simulink model "TrqBasedOnEfficient"  (R2022b)
settings: Solver=VariableStepAuto  StartTime=0.0  StopTime=120  RelTol=1e-3
libraries: Solver_SF x1, simulink x1
settings Model: Creator=12045  LastModifiedBy=12045
settings DebuggingCC: ParameterPrecisionLossMsg=none

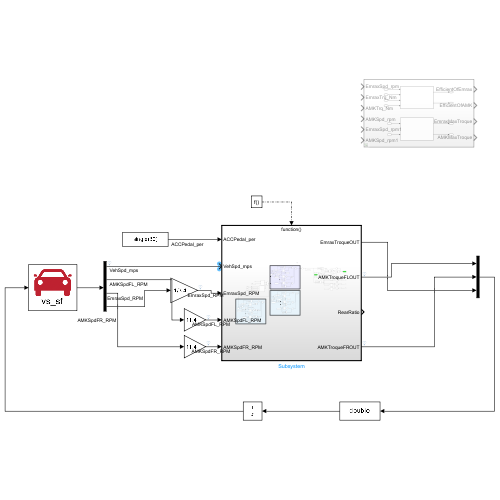
[thumbnail: Simulink's stored preview of the top-level diagram]
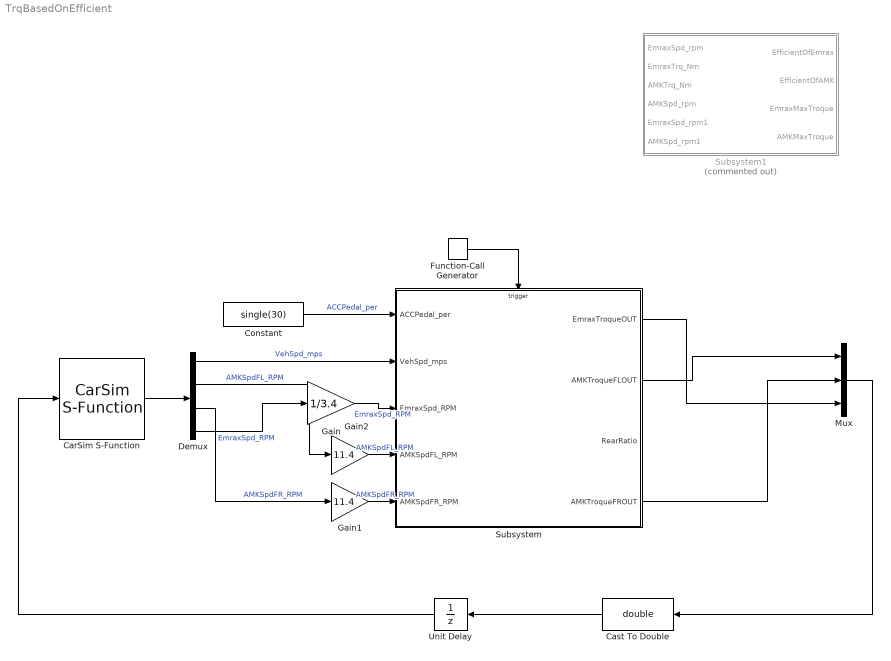
== system TrqBasedOnEfficient ==
  CarSim S-Function : Solver_SF/CarSim S-Function  Priority=1  SIMFILE=simfile.sim  Run_RTs=off  vs_state_ind=Run  StopMode_ind=Vehicle Model
  Cast To Double : DataTypeConversion  OutDataTypeStr=double  SaturateOnIntegerOverflow=off  RndMeth=Floor
  Constant : Constant  Value=single(30)
  Demux : Demux
  Function-Call Generator : simulink/Ports & Subsystems/Function-Call Generator  sample_time=0.01  numberOfIterations=1  DisallowWideOutput=off
  Gain : Gain  Gain=1/3.4
  Gain1 : Gain  Gain=11.4
  Gain2 : Gain  Gain=11.4
  Mux : Mux  Inputs=3
  Subsystem : Subsystem
  Subsystem1 : Subsystem  Commented=on
  Unit Delay : UnitDelay  SampleTime=-1  HasFrameUpgradeWarning=on
  wires:
  Function-Call Generator/1 -> Subsystem/Trigger
  CarSim S-Function/1 -> Demux/1
  Demux/1 -> Subsystem/2(VehSpd_mps)  "VehSpd_mps"
  Demux/2 -> Gain2/1  "AMKSpdFL_RPM"
  Demux/3 -> Gain1/1  "AMKSpdFR_RPM"
  Demux/4 -> Gain/1  "EmraxSpd_RPM"
  Constant/1 -> Subsystem/1(ACCPedal_per)  "ACCPedal_per"
  Subsystem/2(AMKTroqueFLOUT) -> Mux/1
  Subsystem/1(EmraxTroqueOUT) -> Mux/3
  Subsystem/4(AMKTroqueFROUT) -> Mux/2
  Mux/1 -> Cast To Double/1
  Unit Delay/1 -> CarSim S-Function/1
  Cast To Double/1 -> Unit Delay/1
  Gain/1 -> Subsystem/3(EmraxSpd_RPM)  "EmraxSpd_RPM"
  Gain1/1 -> Subsystem/5(AMKSpdFR_RPM)  "AMKSpdFR_RPM"
  Gain2/1 -> Subsystem/4(AMKSpdFL_RPM)  "AMKSpdFL_RPM"

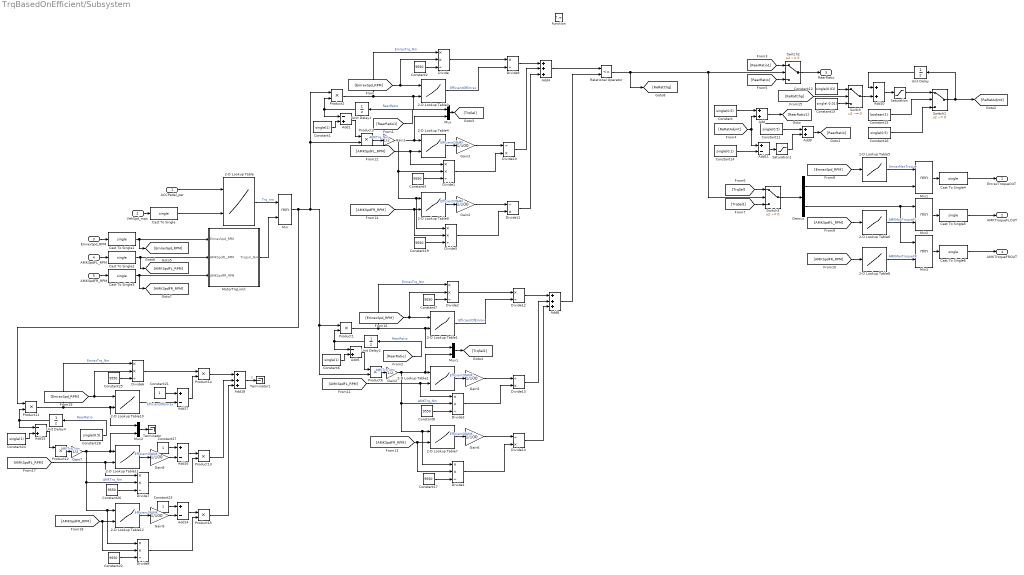
== system TrqBasedOnEfficient/Subsystem ==
  ACCPedal_per : Inport
  VehSpd_mps : Inport  Port=2
  EmraxSpd_RPM : Inport  Port=3
  AMKSpdFL_RPM : Inport  Port=4
  AMKSpdFR_RPM : Inport  Port=5
  function : TriggerPort  TriggerType=function-call  VariantControl=(inherit)
  2-D Lookup Table : Lookup_n-D  BreakpointsForDimension1=single([0 10 20 30 40 50 60 70 80 90 100])  BreakpointsForDimension2=single([5.40000009536743 10.8000001907349 16.2000007629395 21.6000003814697 27 32.4000015258789 37.7999992370605 43.2000007629395 48.5999984741211 54 59.4000015258789 64.8000030517578 70.1999969482422 75.5999984741211 81 86.4000015258789 91.8000030517578 97.1999969482422 102.599998474121 108])  BreakpointsForDimension1DataTypeStr=single  BreakpointsForDimension2DataTypeStr=single  Table=single([0 0 0 0 0 0 0 0 0 0 0 0 0 0 0 0 0 0 0 0;20 20 20 20 20 20 20 18 18 18 17 17 16 16 15 15 15 14 14 14;35 35 35 35 35 35 30 30 25 25 25 25 20 20 20 20 20 20 20 18;50 50 50 50 50 50 50 50 50 40 40 40 40 40 40 40 40 40 38 35;79 79 79 79 85 85 85 90 95 100 110 110 110 100 90 90 80 72 70 65;100 100 100 105 105 105 110 110 110 110 115 115 125 125 120 110 90 80 76 70;120 120 120 120 125 125 125 135 135 135 135 135 135 130 130 120 100 90 82 74;125 125 125 130 135 140 145 155 155 155 155 155 155 155 155 135 110 100 88 82;130 160 160 160 160 170 160 160 160 160 160 160 160 160 160 142 120 105 94 88;130 160 160 160 160 170 160 160 160 160 160 160 160 160 160 142 120 105 95 91;170 170 180 180 180 210 200 200 200 200 200 200 190 180 180 152 133 118 106 100])  InternalRulePriority=Speed  RndMeth=Simplest
      settings: InputPortMap=u0,u1
  2-D Lookup Table1 : Lookup_n-D  BreakpointsForDimension1=[0;200;400;600;800;1000;1200;1400;1600;1800;2000;2200;2400;2600;2800;3000;3200;3400;3600;3800;4000;4200;4400;4600;4800;5000;5200;5400]  BreakpointsForDimension2=[0;25;50;75;100;125;150;175;200;225;250]  Table=[0.7 0.7 0.7 0.7 0.7 0.7 0.7 0.7 0.7 0.7 0.7;0.7 0.7 0.7 0.7 0.7 0.7 0.7 0.7 0.7 0.7 0.7;0.7 0.7 0.86 0.86 0.86 0.86 0.86 0.7 0.7 0.7 0.7;0.7 0.7 0.86 0.86 0.86 0.86 0.86 0.86 0.7 0.7 0.7;0.7 0.82 0.86 0.9 0.9 0.9 0.86 0.86 0.86 0.7 0.7;0.7 0.82 0.86 0.9 0.9 0.9 0.9 0.9 0.86 0.86 0.7;0.7 0.7 0.9 0.94 0.94 0.94 0.94 0.9 0.9 0.86 0.7;0.7 0.82 0.9 0.94 0.94 0.95 0.95 0.94 0.9 0.9 0.7;0.7 0.86 0.9 0.94 0.95 0.95 0.95 0.94 0.9 0.9 0.7;0.7 0.86 0.9 0.94 0.96 0.98 0.95 0.94 0.9 0.9 0.7;0.7 0.86 0.9 0.95 0.96 0.96 0.95 0.94 0.9 0.9 0.7;0.7 0.86 0.9 0.95 0.96 0.96 0.95 0.94 0.94 0.9 0.7;0.7 0.86 0.9 0.95 0.96 0.96 0.95 0.94 0.94 0.9 0.7;0.7 0.86 0.9 0.95 0.96 0.96 0.95 0.94 0.94 0.9 0.7;0.7 0.86 0.9 0.95 0.96 0.96 0.95 0.94 0.94 0.9 0.7;0.7 0.86 0.9 0.95 0.96 0.96 0.95 0.94 0.94 0.9 0.7;0.7 0.86 0.9 0.95 0.96 0.96 0.95 0.94 0.94 0.9 0.7;0.7 0.86 0.9 0.94 0.96 0.96 0.95 0.94 0.94 0.9 0.7;0.7 0.86 0.9 0.94 0.96 0.95 0.95 0.94 0.94 0.9 0.7;0.7 0.86 0.9 0.94 0.96 0.95 0.95 0.94 0.94 0.9 0.7;0.7 0.86 0.9 0.94 0.95 0.95 0.95 0.94 0.94 0.9 0.7;0.7 0.7 0.9 0.94 0.95 0.95 0.95 0.94 0.94 0.9 0.7;0.7 0.7 0.86 0.94 0.94 0.95 0.95 0.94 0.94 0.9 0.7;0.7 0.7 0.86 0.9 0.94 0.95 0.95 0.94 0.94 0.9 0.7;0.7 0.7 0.7 0.9 0.94 0.94 0.94 0.94 0.94 0.9 0.7;0.7 0.7 0.7 0.86 0.9 0.94 0.94 0.94 0.94 0.9 0.7;0.7 0.7 0.7 0.86 0.9 0.9 0.94 0.94 0.94 0.9 0.7;0.7 0.7 0.7 0.86 0.9 0.9 0.94 0.94 0.94 0.9 0.7]  InternalRulePriority=Speed  RndMeth=Simplest
      settings: InputPortMap=u0,u1
  2-D Lookup Table10 : Lookup_n-D  BreakpointsForDimension1=[0;200;400;600;800;1000;1200;1400;1600;1800;2000;2200;2400;2600;2800;3000;3200;3400;3600;3800;4000;4200;4400;4600;4800;5000;5200;5400]  BreakpointsForDimension2=[0;25;50;75;100;125;150;175;200;225;250]  Table=[0.7 0.7 0.7 0.7 0.7 0.7 0.7 0.7 0.7 0.7 0.7;0.7 0.7 0.7 0.7 0.7 0.7 0.7 0.7 0.7 0.7 0.7;0.7 0.7 0.86 0.86 0.86 0.86 0.86 0.7 0.7 0.7 0.7;0.7 0.7 0.86 0.86 0.86 0.86 0.86 0.86 0.7 0.7 0.7;0.7 0.82 0.86 0.9 0.9 0.9 0.86 0.86 0.86 0.7 0.7;0.7 0.82 0.86 0.9 0.9 0.9 0.9 0.9 0.86 0.86 0.7;0.7 0.7 0.9 0.94 0.94 0.94 0.94 0.9 0.9 0.86 0.7;0.7 0.82 0.9 0.94 0.94 0.95 0.95 0.94 0.9 0.9 0.7;0.7 0.86 0.9 0.94 0.95 0.95 0.95 0.94 0.9 0.9 0.7;0.7 0.86 0.9 0.94 0.96 0.98 0.95 0.94 0.9 0.9 0.7;0.7 0.86 0.9 0.95 0.96 0.96 0.95 0.94 0.9 0.9 0.7;0.7 0.86 0.9 0.95 0.96 0.96 0.95 0.94 0.94 0.9 0.7;0.7 0.86 0.9 0.95 0.96 0.96 0.95 0.94 0.94 0.9 0.7;0.7 0.86 0.9 0.95 0.96 0.96 0.95 0.94 0.94 0.9 0.7;0.7 0.86 0.9 0.95 0.96 0.96 0.95 0.94 0.94 0.9 0.7;0.7 0.86 0.9 0.95 0.96 0.96 0.95 0.94 0.94 0.9 0.7;0.7 0.86 0.9 0.95 0.96 0.96 0.95 0.94 0.94 0.9 0.7;0.7 0.86 0.9 0.94 0.96 0.96 0.95 0.94 0.94 0.9 0.7;0.7 0.86 0.9 0.94 0.96 0.95 0.95 0.94 0.94 0.9 0.7;0.7 0.86 0.9 0.94 0.96 0.95 0.95 0.94 0.94 0.9 0.7;0.7 0.86 0.9 0.94 0.95 0.95 0.95 0.94 0.94 0.9 0.7;0.7 0.7 0.9 0.94 0.95 0.95 0.95 0.94 0.94 0.9 0.7;0.7 0.7 0.86 0.94 0.94 0.95 0.95 0.94 0.94 0.9 0.7;0.7 0.7 0.86 0.9 0.94 0.95 0.95 0.94 0.94 0.9 0.7;0.7 0.7 0.7 0.9 0.94 0.94 0.94 0.94 0.94 0.9 0.7;0.7 0.7 0.7 0.86 0.9 0.94 0.94 0.94 0.94 0.9 0.7;0.7 0.7 0.7 0.86 0.9 0.9 0.94 0.94 0.94 0.9 0.7;0.7 0.7 0.7 0.86 0.9 0.9 0.94 0.94 0.94 0.9 0.7]  InternalRulePriority=Speed  RndMeth=Simplest
      settings: InputPortMap=u0,u1
  2-D Lookup Table{2,4,7,9,11..12} (6 alike) : Lookup_n-D  BreakpointsForDimension1=[1.3;2.7;5.4;7.9;10.4;12.5;14.4;16;17.4;18.5;19.6]  BreakpointsForDimension2=[500;1000;2000;3000;4000;6000;10000;12000;15000;19000]  Table=[64.37 71.33 73.64 74.7 75.43 76.57 77 77.08 77.56 78.14;58.42 70.48 77.57 80.4 82.01 83.92 85.16 85.44 85.97 86.5;44.94 60.81 73.35 78.82 81.94 85.43 88.2 88.88 89.71 90.44;35.59 51.9 67.02 74.26 78.54 83.42 87.58 88.65 89.84 90.86;29.14 44.78 61.01 69.41 74.57 80.62 85.93 87.34 88.86 90.16;24.17 38.71 55.22 64.39 70.24 77.3 83.73 85.48 87.37 88.98;20.41 33.76 50.04 59.65 65.99 73.88 81.33 83.42 85.66 87.59;17.31 29.4 45.1 54.87 61.55 70.1 78.56 80.97 83.56 85.81;14.82 25.75 40.67 50.41 57.28 66.34 75.7 78.4 81.34 83.91;12.81 22.67 36.72 46.3 53.25 62.67 72.77 75.75 79.02 81.91;11.17 20.05 33.21 42.51 49.44 59.09 69.82 73.06 76.63 79.83]  InternalRulePriority=Speed  RndMeth=Simplest
      settings: InputPortMap=u0,u1
  2-D Lookup Table3 : Lookup_n-D  BreakpointsForDimension1=[0;200;400;600;800;1000;1200;1400;1600;1800;2000;2200;2400;2600;2800;3000;3200;3400;3600;3800;4000;4200;4400;4600;4800;5000;5200;5400]  BreakpointsForDimension2=[0;25;50;75;100;125;150;175;200;225;250]  Table=[0.7 0.7 0.7 0.7 0.7 0.7 0.7 0.7 0.7 0.7 0.7;0.7 0.7 0.7 0.7 0.7 0.7 0.7 0.7 0.7 0.7 0.7;0.7 0.7 0.86 0.86 0.86 0.86 0.86 0.7 0.7 0.7 0.7;0.7 0.7 0.86 0.86 0.86 0.86 0.86 0.86 0.7 0.7 0.7;0.7 0.82 0.86 0.9 0.9 0.9 0.86 0.86 0.86 0.7 0.7;0.7 0.82 0.86 0.9 0.9 0.9 0.9 0.9 0.86 0.86 0.7;0.7 0.7 0.9 0.94 0.94 0.94 0.94 0.9 0.9 0.86 0.7;0.7 0.82 0.9 0.94 0.94 0.95 0.95 0.94 0.9 0.9 0.7;0.7 0.86 0.9 0.94 0.95 0.95 0.95 0.94 0.9 0.9 0.7;0.7 0.86 0.9 0.94 0.96 0.98 0.95 0.94 0.9 0.9 0.7;0.7 0.86 0.9 0.95 0.96 0.96 0.95 0.94 0.9 0.9 0.7;0.7 0.86 0.9 0.95 0.96 0.96 0.95 0.94 0.94 0.9 0.7;0.7 0.86 0.9 0.95 0.96 0.96 0.95 0.94 0.94 0.9 0.7;0.7 0.86 0.9 0.95 0.96 0.96 0.95 0.94 0.94 0.9 0.7;0.7 0.86 0.9 0.95 0.96 0.96 0.95 0.94 0.94 0.9 0.7;0.7 0.86 0.9 0.95 0.96 0.96 0.95 0.94 0.94 0.9 0.7;0.7 0.86 0.9 0.95 0.96 0.96 0.95 0.94 0.94 0.9 0.7;0.7 0.86 0.9 0.94 0.96 0.96 0.95 0.94 0.94 0.9 0.7;0.7 0.86 0.9 0.94 0.96 0.95 0.95 0.94 0.94 0.9 0.7;0.7 0.86 0.9 0.94 0.96 0.95 0.95 0.94 0.94 0.9 0.7;0.7 0.86 0.9 0.94 0.95 0.95 0.95 0.94 0.94 0.9 0.7;0.7 0.7 0.9 0.94 0.95 0.95 0.95 0.94 0.94 0.9 0.7;0.7 0.7 0.86 0.94 0.94 0.95 0.95 0.94 0.94 0.9 0.7;0.7 0.7 0.86 0.9 0.94 0.95 0.95 0.94 0.94 0.9 0.7;0.7 0.7 0.7 0.9 0.94 0.94 0.94 0.94 0.94 0.9 0.7;0.7 0.7 0.7 0.86 0.9 0.94 0.94 0.94 0.94 0.9 0.7;0.7 0.7 0.7 0.86 0.9 0.9 0.94 0.94 0.94 0.9 0.7;0.7 0.7 0.7 0.86 0.9 0.9 0.94 0.94 0.94 0.9 0.7]  InternalRulePriority=Speed  RndMeth=Simplest
      settings: InputPortMap=u0,u1
  2-D Lookup Table5 : Lookup_n-D  NumberOfTableDimensions=1  BreakpointsForDimension1=[200;400;600;800;1000;1200;1400;1600;1800;2000;2200;2400;2600;2800;3000;3200;3400;3600;3800;4000;4200;4400;4600;4800;5000;5200;5400]  BreakpointsForDimension2=[1:3]  Table=[229.85;229.85;229.85;229.85;229.85;229.85;229.85;229.85;229.85;229.85;229.85;229.85;229.46;229.16;228.86;228.86;228.86;228.86;228.86;227.86;227.86;226.87;225.86;224.86;220.86;218.87;215.87]  InternalRulePriority=Speed  RndMeth=Simplest
  2-D Lookup Table6 : Lookup_n-D  NumberOfTableDimensions=1  BreakpointsForDimension1=[0;1000;2000;3000;4000;5000;6000;7000;8000;9000;10000;11000;12000;13000;14000;15000;16000;17000;18000;19000]  BreakpointsForDimension2=[1:3]  Table=[21;21;21;21;21;21;21;21;21;21;21;21;21;21;20;17.5;15;12.5;8;0]  InternalRulePriority=Speed  RndMeth=Simplest
  2-D Lookup Table8 : Lookup_n-D  NumberOfTableDimensions=1  BreakpointsForDimension1=[0;1000;2000;3000;4000;5000;6000;7000;8000;9000;10000;11000;12000;13000;14000;15000;16000;17000;18000;19000]  BreakpointsForDimension2=[1:3]  Table=[21;21;21;21;21;21;21;21;21;21;21;21;21;21;20;17.5;15;12.5;8;0]  InternalRulePriority=Speed  RndMeth=Simplest
  Add : Sum
  Add1 : Sum  Inputs=-+
  Add10 : Sum
  Add{11,14,16..17} (4 alike) : Sum  Inputs=+-
  Add15 : Sum  Inputs=-+
  Add18 : Sum  Inputs=+++
  Add4 : Sum  Inputs=+++
  Add5 : Sum  Inputs=-+
  Add8 : Sum  Inputs=+++
  Add9 : Sum
  Cast To Single{,1..6} (7 alike) : DataTypeConversion  OutDataTypeStr=single  SaturateOnIntegerOverflow=off  RndMeth=Floor
  Constant{,11,16,28} (4 alike) : Constant  Value=single(0.5)
  Constant1 : Constant  Value=single(1)
  Constant12 : Constant  Value=single(0.01)
  Constant13 : Constant  Value=single(-0.01)
  Constant14 : Constant  Value=single(0.1)
  Constant15 : Constant  Value=boolean(1)
  Constant{2..3,7..8,17,19,22,25..26} (9 alike) : Constant  Value=9550
  Constant21 : Constant
  Constant23 : Constant
  Constant24 : Constant  Value=single(1)
  Constant27 : Constant
  Constant6 : Constant  Value=single(1)
  Demux : Demux  Outputs=2
  Divide{,1..8} (9 alike) : Product  Inputs=**/
  Divide{10..11,13..14} (4 alike) : Product  Inputs=/*
  Divide12 : Product  Inputs=*/
  Divide9 : Product  Inputs=*/
  Gain1 : Gain  Gain=1/2
  Gain2 : Gain  Gain=1/2
  Gain{3..6,8..9} (6 alike) : Gain  Gain=1/100
  Gain7 : Gain  Gain=1/2
  Min{,1..3} (4 alike) : MinMax  Inputs=2
  MotorTrqLimit : Subsystem
  Mux : Mux  Inputs=2
  Mux1 : Mux  Inputs=2
  Mux2 : Mux  Inputs=2
  Product{1..3,6,11..15} (9 alike) : Product
  Relational Operator : RelationalOperator  Operator=<=  OutDataTypeStr=boolean  RndMeth=Simplest  InputSameDT=off
  Saturation : Saturate  LowerLimit=0
  Saturation1 : Saturate  UpperLimit=1  LowerLimit=0.5
  Switch{,1..3} (4 alike) : Switch  Criteria=u2 ~= 0  SaturateOnIntegerOverflow=off  InputSameDT=off
  Terminator : Terminator
  Terminator1 : Terminator
  Unit Delay : UnitDelay  SampleTime=-1  HasFrameUpgradeWarning=on
  Unit Delay1 : UnitDelay  InitialCondition=0.5  SampleTime=-1  HasFrameUpgradeWarning=on
  Unit Delay2 : UnitDelay  InitialCondition=0.5  SampleTime=-1  HasFrameUpgradeWarning=on
  Unit Delay4 : UnitDelay  InitialCondition=0.5  SampleTime=-1  HasFrameUpgradeWarning=on
  EmraxTroqueOUT : Outport
  AMKTroqueFLOUT : Outport  Port=2
  RearRatio : Outport  Port=3
  AMKTroqueFROUT : Outport  Port=4
  wires:
  2-D Lookup Table/1 -> Min/1  "Trq_nm"
  MotorTrqLimit/1(TrqLim_Nm) -> Min/2
  2-D Lookup Table6/1 -> Min2/2  "AMKMaxTroqueFL"
  [EmraxSpd_RPM] -> 2-D Lookup Table5/1
  [AMKSpdFL_RPM] -> 2-D Lookup Table6/1
  2-D Lookup Table5/1 -> Min1/1  "EmraxMaxTroque"
  ACCPedal_per/1 -> 2-D Lookup Table/1
  EmraxSpd_RPM/1 -> Cast To Single1/1
  VehSpd_mps/1 -> Cast To Single/1
  Unit Delay1/1 -> Add1/1, Product2/2
  [AMKSpdFL_RPM] -> Divide1/1, 2-D Lookup Table4/2
  [EmraxSpd_RPM] -> Divide/2, 2-D Lookup Table3/1
  2-D Lookup Table4/1 -> Gain3/1  "EfficientOfAMK"
  2-D Lookup Table3/1 -> Divide9/2  "EfficientOfEmrax"
  Constant1/1 -> Add1/2
  Product3/1 -> Gain1/1  "AMKTrq_Nm"
  [RearRatio1] -> Unit Delay1/1  "RearRatio"
  Add1/1 -> Product3/1
  Min/1 -> Product11/1, Product6/2, Product1/1, Product2/1, Product3/2
  Product2/1 -> Divide/1, Mux/1, 2-D Lookup Table3/2  "EmraxTrq_Nm"
  Constant2/1 -> Divide/3
  Constant3/1 -> Divide1/3
  Divide1/1 -> Divide10/2
  Divide/1 -> Divide9/1
  Divide9/1 -> Add4/1
  Divide10/1 -> Add4/2
  Divide13/1 -> Add8/2
  Divide12/1 -> Add8/1
  Divide2/1 -> Divide12/1
  Constant8/1 -> Divide3/3
  Constant7/1 -> Divide2/3
  Product1/1 -> Mux1/1, 2-D Lookup Table1/2, Divide2/1  "EmraxTrq_Nm"
  Add5/1 -> Product6/1
  [RearRatio] -> Unit Delay2/1  "RearRatio"
  Gain2/1 -> Mux1/2, 2-D Lookup Table2/1, Divide3/2, Divide4/1, 2-D Lookup Table7/1  "AMKTrq_Nm"
  Constant6/1 -> Add5/2
  2-D Lookup Table1/1 -> Divide12/2  "EfficientOfEmrax"
  2-D Lookup Table2/1 -> Gain5/1  "EfficientOfAMK"
  [EmraxSpd_RPM] -> 2-D Lookup Table1/1, Divide2/2
  [AMKSpdFL_RPM] -> 2-D Lookup Table2/2, Divide3/1
  Unit Delay2/1 -> Product1/2, Add5/1
  Constant/1 -> Add/1
  Constant11/1 -> Add9/1
  Add/1 -> [RearRatio1]
  Add9/1 -> [RearRatio]
  Add4/1 -> Relational Operator/1
  Constant12/1 -> Switch/1
  Constant13/1 -> Switch/3
  Switch/1 -> Add10/2
  Add10/1 -> Saturation/1
  Switch1/1 -> [ReRatAdjmt], Unit Delay/1
  Unit Delay/1 -> Add10/1
  Saturation/1 -> Switch1/1
  Constant15/1 -> Switch1/2
  Add8/1 -> Relational Operator/2
  [ReRatAdjmt] -> Add/2, Add11/1
  Add11/1 -> Saturation1/1
  Constant14/1 -> Add11/2
  Saturation1/1 -> Add9/2
  [RearRatio1] -> Switch2/1
  [RearRatio] -> Switch2/3
  Switch2/1 -> RearRatio/1
  Constant16/1 -> Switch1/3
  AMKSpdFL_RPM/1 -> Cast To Single2/1
  Cast To Single/1 -> 2-D Lookup Table/2
  Mux/1 -> [TrqSel]
  Mux1/1 -> [TrqSel1]
  [TrqSel] -> Switch3/1
  [TrqSel1] -> Switch3/3
  Switch3/1 -> Demux/1
  AMKSpdFR_RPM/1 -> Cast To Single3/1
  [AMKSpdFR_RPM] -> 2-D Lookup Table8/1
  2-D Lookup Table8/1 -> Min3/2  "AMKMaxTroqueFR"
  Product6/1 -> Gain2/1  "AMKTrq_Nm"
  Gain1/1 -> 2-D Lookup Table4/1, Mux/2, Divide1/2, Divide5/1, 2-D Lookup Table9/1
  [AMKSpdFR_RPM] -> Divide4/2, 2-D Lookup Table7/2
  [AMKSpdFR_RPM] -> Divide5/2, 2-D Lookup Table9/2
  Constant17/1 -> Divide4/3
  2-D Lookup Table7/1 -> Gain6/1  "EfficientOfAMK"
  Divide4/1 -> Divide14/2
  Divide14/1 -> Add8/3
  Constant19/1 -> Divide5/3
  Divide5/1 -> Divide11/2
  2-D Lookup Table9/1 -> Gain4/1  "EfficientOfAMK"
  Divide11/1 -> Add4/3
  Cast To Single1/1 -> MotorTrqLimit/1(EmraxSpd_RPM), [EmraxSpd_RPM]
  Cast To Single2/1 -> MotorTrqLimit/2(AMKSpdFL_RPM), [AMKSpdFL_RPM]
  Cast To Single3/1 -> [AMKSpdFR_RPM], MotorTrqLimit/3(AMKSpdFR_RPM)
  Demux/1 -> Min1/2
  Demux/2 -> Min3/1, Min2/1
  Min1/1 -> Cast To Single4/1
  Min2/1 -> Cast To Single5/1
  Min3/1 -> Cast To Single6/1
  [ReRatChg] -> Switch/2
  Cast To Single4/1 -> EmraxTroqueOUT/1
  Cast To Single5/1 -> AMKTroqueFLOUT/1
  Cast To Single6/1 -> AMKTroqueFROUT/1
  Gain3/1 -> Divide10/1
  Gain4/1 -> Divide11/1
  Gain5/1 -> Divide13/1
  Gain6/1 -> Divide14/1
  Gain9/1 -> Add14/2
  Gain8/1 -> Add16/2
  Product15/1 -> Add18/3
  Divide8/1 -> Product15/2
  Add14/1 -> Product15/1
  Constant23/1 -> Add14/1
  2-D Lookup Table12/1 -> Gain9/1  "EfficientOfAMK"
  Constant22/1 -> Divide8/3
  [AMKSpdFR_RPM] -> 2-D Lookup Table12/2, Divide8/2
  Product12/1 -> Gain7/1  "AMKTrq_Nm"
  Mux2/1 -> Terminator/1
  Unit Delay4/1 -> Add15/1, Product11/2
  [AMKSpdFL_RPM] -> Divide7/1, 2-D Lookup Table11/2
  [EmraxSpd_RPM] -> Divide6/2, 2-D Lookup Table10/1
  2-D Lookup Table11/1 -> Gain8/1  "EfficientOfAMK"
  2-D Lookup Table10/1 -> Add17/2  "EfficientOfEmrax"
  Constant24/1 -> Add15/2
  Gain7/1 -> 2-D Lookup Table12/1, Divide8/1, Divide7/2, 2-D Lookup Table11/1, Mux2/2  "AMKTrq_Nm"
  Constant28/1 -> Unit Delay4/1  "RearRatio"
  Add15/1 -> Product12/1
  Product11/1 -> Divide6/1, 2-D Lookup Table10/2, Mux2/1  "EmraxTrq_Nm"
  Constant25/1 -> Divide6/3
  Constant26/1 -> Divide7/3
  Constant27/1 -> Add16/1
  Add16/1 -> Product13/1
  Divide7/1 -> Product13/2
  Constant21/1 -> Add17/1
  Divide6/1 -> Product14/1
  Add17/1 -> Product14/2
  Product14/1 -> Add18/1
  Product13/1 -> Add18/2
  Add18/1 -> Terminator1/1  "1"
  Relational Operator/1 -> [ReRatChg], Switch2/2, Switch3/2
  Divide3/1 -> Divide13/2

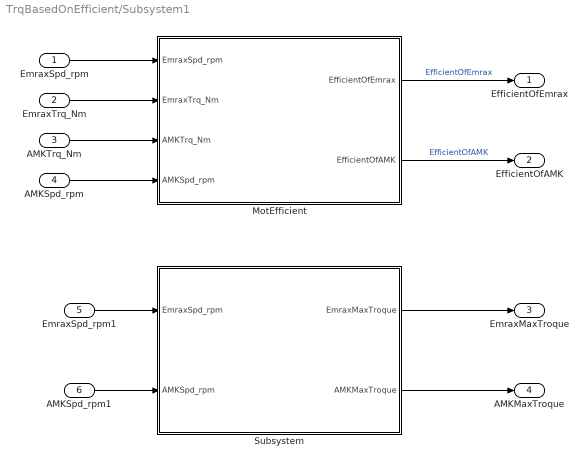
== system TrqBasedOnEfficient/Subsystem1 ==
  EmraxSpd_rpm : Inport
  EmraxTrq_Nm : Inport  Port=2
  AMKTrq_Nm : Inport  Port=3
  AMKSpd_rpm : Inport  Port=4
  EmraxSpd_rpm1 : Inport  Port=5
  AMKSpd_rpm1 : Inport  Port=6
  MotEfficient : Subsystem
  Subsystem : Subsystem
  EfficientOfEmrax : Outport
  EfficientOfAMK : Outport  Port=2
  EmraxMaxTroque : Outport  Port=3
  AMKMaxTroque : Outport  Port=4
  wires:
  MotEfficient/2(EfficientOfAMK) -> EfficientOfAMK/1  "EfficientOfAMK"
  MotEfficient/1(EfficientOfEmrax) -> EfficientOfEmrax/1  "EfficientOfEmrax"
  Subsystem/1(EmraxMaxTroque) -> EmraxMaxTroque/1
  AMKSpd_rpm/1 -> MotEfficient/4(AMKSpd_rpm)
  EmraxSpd_rpm1/1 -> Subsystem/1(EmraxSpd_rpm)
  Subsystem/2(AMKMaxTroque) -> AMKMaxTroque/1
  AMKTrq_Nm/1 -> MotEfficient/3(AMKTrq_Nm)
  EmraxTrq_Nm/1 -> MotEfficient/2(EmraxTrq_Nm)
  EmraxSpd_rpm/1 -> MotEfficient/1(EmraxSpd_rpm)
  AMKSpd_rpm1/1 -> Subsystem/2(AMKSpd_rpm)

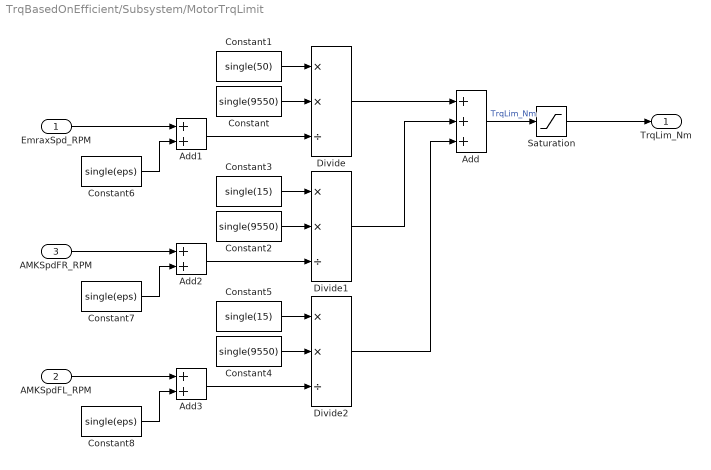
== system TrqBasedOnEfficient/Subsystem/MotorTrqLimit ==
  EmraxSpd_RPM : Inport
  AMKSpdFL_RPM : Inport  Port=2
  AMKSpdFR_RPM : Inport  Port=3
  Add : Sum  Inputs=+++
  Add1 : Sum
  Add2 : Sum
  Add3 : Sum
  Constant : Constant  Value=single(9550)
  Constant1 : Constant  Value=single(50)
  Constant2 : Constant  Value=single(9550)
  Constant3 : Constant  Value=single(15)
  Constant4 : Constant  Value=single(9550)
  Constant5 : Constant  Value=single(15)
  Constant6 : Constant  Value=single(eps)
  Constant7 : Constant  Value=single(eps)
  Constant8 : Constant  Value=single(eps)
  Divide : Product  Inputs=**/
  Divide1 : Product  Inputs=**/
  Divide2 : Product  Inputs=**/
  Saturation : Saturate  UpperLimit=180  LowerLimit=0
  TrqLim_Nm : Outport
  wires:
  Add/1 -> Saturation/1  "TrqLim_Nm"
  EmraxSpd_RPM/1 -> Add1/1
  Constant/1 -> Divide/2
  Constant1/1 -> Divide/1
  Constant3/1 -> Divide1/1
  Constant2/1 -> Divide1/2
  AMKSpdFR_RPM/1 -> Add2/1
  AMKSpdFL_RPM/1 -> Add3/1
  Constant4/1 -> Divide2/2
  Constant5/1 -> Divide2/1
  Divide/1 -> Add/1
  Divide1/1 -> Add/2
  Divide2/1 -> Add/3
  Saturation/1 -> TrqLim_Nm/1
  Add1/1 -> Divide/3
  Constant6/1 -> Add1/2
  Add2/1 -> Divide1/3
  Constant7/1 -> Add2/2
  Add3/1 -> Divide2/3
  Constant8/1 -> Add3/2

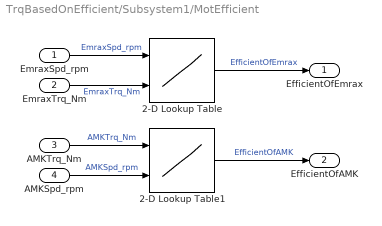
== system TrqBasedOnEfficient/Subsystem1/MotEfficient ==
  EmraxSpd_rpm : Inport
  EmraxTrq_Nm : Inport  Port=2
  AMKTrq_Nm : Inport  Port=3
  AMKSpd_rpm : Inport  Port=4
  2-D Lookup Table : Lookup_n-D  BreakpointsForDimension1=[0;200;400;600;800;1000;1200;1400;1600;1800;2000;2200;2400;2600;2800;3000;3200;3400;3600;3800;4000;4200;4400;4600;4800;5000;5200;5400]  BreakpointsForDimension2=[0;25;50;75;100;125;150;175;200;225;250]  Table=[0.7 0.7 0.7 0.7 0.7 0.7 0.7 0.7 0.7 0.7 0.7;0.7 0.7 0.7 0.7 0.7 0.7 0.7 0.7 0.7 0.7 0.7;0.7 0.7 0.86 0.86 0.86 0.86 0.86 0.7 0.7 0.7 0.7;0.7 0.7 0.86 0.86 0.86 0.86 0.86 0.86 0.7 0.7 0.7;0.7 0.82 0.86 0.9 0.9 0.9 0.86 0.86 0.86 0.7 0.7;0.7 0.82 0.86 0.9 0.9 0.9 0.9 0.9 0.86 0.86 0.7;0.7 0.7 0.9 0.94 0.94 0.94 0.94 0.9 0.9 0.86 0.7;0.7 0.82 0.9 0.94 0.94 0.95 0.95 0.94 0.9 0.9 0.7;0.7 0.86 0.9 0.94 0.95 0.95 0.95 0.94 0.9 0.9 0.7;0.7 0.86 0.9 0.94 0.96 0.98 0.95 0.94 0.9 0.9 0.7;0.7 0.86 0.9 0.95 0.96 0.96 0.95 0.94 0.9 0.9 0.7;0.7 0.86 0.9 0.95 0.96 0.96 0.95 0.94 0.94 0.9 0.7;0.7 0.86 0.9 0.95 0.96 0.96 0.95 0.94 0.94 0.9 0.7;0.7 0.86 0.9 0.95 0.96 0.96 0.95 0.94 0.94 0.9 0.7;0.7 0.86 0.9 0.95 0.96 0.96 0.95 0.94 0.94 0.9 0.7;0.7 0.86 0.9 0.95 0.96 0.96 0.95 0.94 0.94 0.9 0.7;0.7 0.86 0.9 0.95 0.96 0.96 0.95 0.94 0.94 0.9 0.7;0.7 0.86 0.9 0.94 0.96 0.96 0.95 0.94 0.94 0.9 0.7;0.7 0.86 0.9 0.94 0.96 0.95 0.95 0.94 0.94 0.9 0.7;0.7 0.86 0.9 0.94 0.96 0.95 0.95 0.94 0.94 0.9 0.7;0.7 0.86 0.9 0.94 0.95 0.95 0.95 0.94 0.94 0.9 0.7;0.7 0.7 0.9 0.94 0.95 0.95 0.95 0.94 0.94 0.9 0.7;0.7 0.7 0.86 0.94 0.94 0.95 0.95 0.94 0.94 0.9 0.7;0.7 0.7 0.86 0.9 0.94 0.95 0.95 0.94 0.94 0.9 0.7;0.7 0.7 0.7 0.9 0.94 0.94 0.94 0.94 0.94 0.9 0.7;0.7 0.7 0.7 0.86 0.9 0.94 0.94 0.94 0.94 0.9 0.7;0.7 0.7 0.7 0.86 0.9 0.9 0.94 0.94 0.94 0.9 0.7;0.7 0.7 0.7 0.86 0.9 0.9 0.94 0.94 0.94 0.9 0.7]  InternalRulePriority=Speed  RndMeth=Simplest
      settings: InputPortMap=u0,u1
  2-D Lookup Table1 : Lookup_n-D  BreakpointsForDimension1=[1.3;2.7;5.4;7.9;10.4;12.5;14.4;16;17.4;18.5;19.6]  BreakpointsForDimension2=[500;1000;2000;3000;4000;6000;10000;12000;15000;19000]  Table=[64.37 71.33 73.64 74.7 75.43 76.57 77 77.08 77.56 78.14;58.42 70.48 77.57 80.4 82.01 83.92 85.16 85.44 85.97 86.5;44.94 60.81 73.35 78.82 81.94 85.43 88.2 88.88 89.71 90.44;35.59 51.9 67.02 74.26 78.54 83.42 87.58 88.65 89.84 90.86;29.14 44.78 61.01 69.41 74.57 80.62 85.93 87.34 88.86 90.16;24.17 38.71 55.22 64.39 70.24 77.3 83.73 85.48 87.37 88.98;20.41 33.76 50.04 59.65 65.99 73.88 81.33 83.42 85.66 87.59;17.31 29.4 45.1 54.87 61.55 70.1 78.56 80.97 83.56 85.81;14.82 25.75 40.67 50.41 57.28 66.34 75.7 78.4 81.34 83.91;12.81 22.67 36.72 46.3 53.25 62.67 72.77 75.75 79.02 81.91;11.17 20.05 33.21 42.51 49.44 59.09 69.82 73.06 76.63 79.83]  InternalRulePriority=Speed  RndMeth=Simplest
      settings: InputPortMap=u0,u1
  EfficientOfEmrax : Outport
  EfficientOfAMK : Outport  Port=2
  wires:
  EmraxSpd_rpm/1 -> 2-D Lookup Table/1  "EmraxSpd_rpm"
  AMKTrq_Nm/1 -> 2-D Lookup Table1/1  "AMKTrq_Nm"
  AMKSpd_rpm/1 -> 2-D Lookup Table1/2  "AMKSpd_rpm"
  EmraxTrq_Nm/1 -> 2-D Lookup Table/2  "EmraxTrq_Nm"
  2-D Lookup Table1/1 -> EfficientOfAMK/1  "EfficientOfAMK"
  2-D Lookup Table/1 -> EfficientOfEmrax/1  "EfficientOfEmrax"

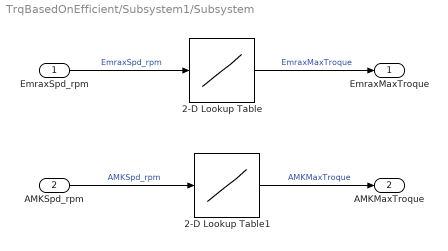
== system TrqBasedOnEfficient/Subsystem1/Subsystem ==
  EmraxSpd_rpm : Inport
  AMKSpd_rpm : Inport  Port=2
  2-D Lookup Table : Lookup_n-D  NumberOfTableDimensions=1  BreakpointsForDimension1=[200;400;600;800;1000;1200;1400;1600;1800;2000;2200;2400;2600;2800;3000;3200;3400;3600;3800;4000;4200;4400;4600;4800;5000;5200;5400]  BreakpointsForDimension2=[1:3]  Table=[229.85;229.85;229.85;229.85;229.85;229.85;229.85;229.85;229.85;229.85;229.85;229.85;229.46;229.16;228.86;228.86;228.86;228.86;228.86;227.86;227.86;226.87;225.86;224.86;220.86;218.87;215.87]  InternalRulePriority=Speed  RndMeth=Simplest
  2-D Lookup Table1 : Lookup_n-D  NumberOfTableDimensions=1  BreakpointsForDimension1=[0;1000;2000;3000;4000;5000;6000;7000;8000;9000;10000;11000;12000;13000;14000;15000;16000;17000;18000;19000]  BreakpointsForDimension2=[1:3]  Table=[21;21;21;21;21;21;21;21;21;21;21;21;21;21;20;17.5;15;12.5;8;0]  InternalRulePriority=Speed  RndMeth=Simplest
  EmraxMaxTroque : Outport
  AMKMaxTroque : Outport  Port=2
  wires:
  EmraxSpd_rpm/1 -> 2-D Lookup Table/1  "EmraxSpd_rpm"
  2-D Lookup Table/1 -> EmraxMaxTroque/1  "EmraxMaxTroque"
  AMKSpd_rpm/1 -> 2-D Lookup Table1/1  "AMKSpd_rpm"
  2-D Lookup Table1/1 -> AMKMaxTroque/1  "AMKMaxTroque"
